simulink model "Gain_test"  (R2022a)
settings: Solver=VariableStepAuto  StartTime=0.0  StopTime=10.0  RelTol=1e-3
settings Model: Creator=Martin  LastModifiedBy=Martin

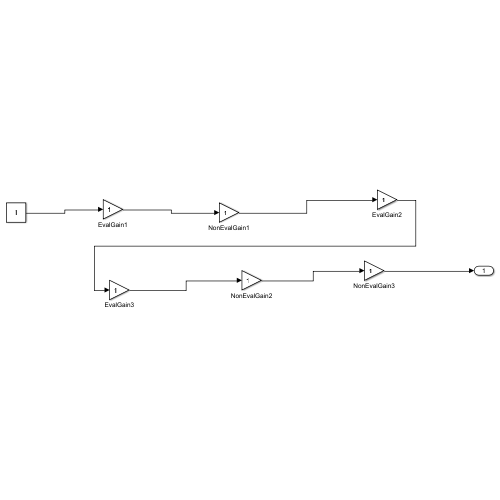
[thumbnail: Simulink's stored preview of the top-level diagram]
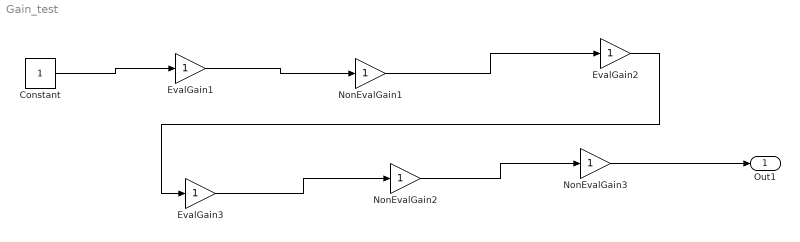
== system Gain_test ==
  Constant : Constant
  EvalGain1 : Gain
  EvalGain2 : Gain
  EvalGain3 : Gain
  NonEvalGain1 : Gain
  NonEvalGain2 : Gain
  NonEvalGain3 : Gain
  Out1 : Outport
  wires:
  EvalGain1/1 -> NonEvalGain1/1
  NonEvalGain1/1 -> EvalGain2/1
  EvalGain2/1 -> EvalGain3/1
  EvalGain3/1 -> NonEvalGain2/1
  NonEvalGain2/1 -> NonEvalGain3/1
  Constant/1 -> EvalGain1/1
  NonEvalGain3/1 -> Out1/1
